simulink model "Vergleich_linear_nichtlinear"  (R2021b)
settings: Solver=FixedStepAuto  StartTime=0.0  StopTime=25  FixedStep=1/1e4  RelTol=1e-3
undefined symbols (not defined in the file): A, B, C, D, S, T_c
settings Model: Creator=basti  LastModifiedBy=basti

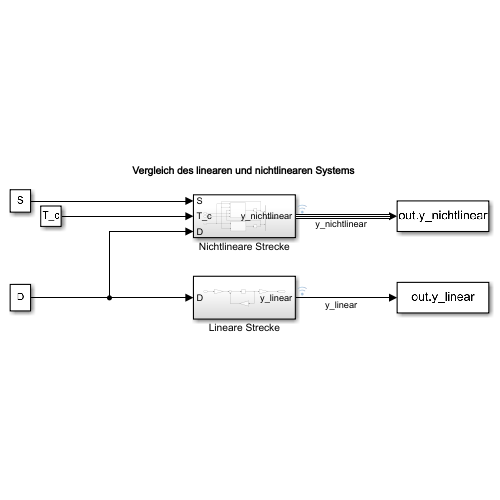
[thumbnail: Simulink's stored preview of the top-level diagram]
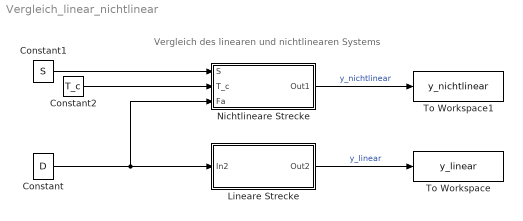
== system Vergleich_linear_nichtlinear ==
  note: Vergleich des linearen und nichtlinearen Systems
  Constant : Constant  Value=D
  Constant1 : Constant  Value=S
  Constant2 : Constant  Value=T_c
  Lineare Strecke : Subsystem
  Nichtlineare Strecke : Subsystem
  To Workspace : ToWorkspace  VariableName=y_linear  SaveFormat=Timeseries  SampleTime=-1
  To Workspace1 : ToWorkspace  VariableName=y_nichtlinear  SaveFormat=Timeseries  SampleTime=-1
  wires:
  Nichtlineare Strecke/1(Out1) -> To Workspace1/1  "y_nichtlinear"
  Lineare Strecke/1(Out2) -> To Workspace/1  "y_linear"
  Constant/1 -> Lineare Strecke/1(In2), Nichtlineare Strecke/3(Fa)
  Constant1/1 -> Nichtlineare Strecke/1(S)
  Constant2/1 -> Nichtlineare Strecke/2(T_c)

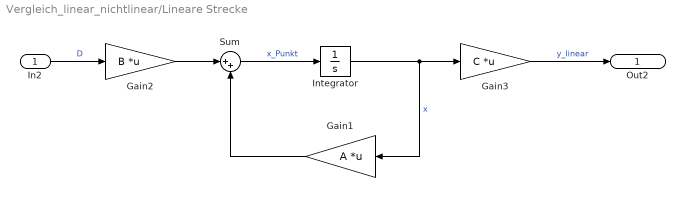
== system Vergleich_linear_nichtlinear/Lineare Strecke ==
  In2 : Inport
  Gain1 : Gain  Gain=A  Multiplication=Matrix(K*u) (u vector)
  Gain2 : Gain  Gain=B  Multiplication=Matrix(K*u) (u vector)
  Gain3 : Gain  Gain=C  Multiplication=Matrix(K*u) (u vector)
  Integrator : Integrator
  Sum : Sum  Inputs=|++
  Out2 : Outport
  wires:
  In2/1 -> Gain2/1  "D"
  Gain2/1 -> Sum/1
  Gain1/1 -> Sum/2
  Sum/1 -> Integrator/1  "x_Punkt"
  Integrator/1 -> Gain3/1, Gain1/1  "x"
  Gain3/1 -> Out2/1  "y_linear"

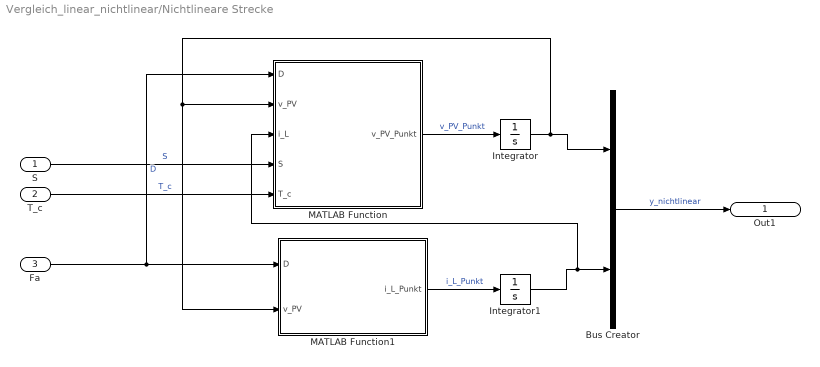
== system Vergleich_linear_nichtlinear/Nichtlineare Strecke ==
  S : Inport
  T_c : Inport  Port=2
  Fa : Inport  Port=3
  Bus Creator : BusCreator  Inputs=2
  Integrator : Integrator
  Integrator1 : Integrator
  MATLAB Function : MATLAB Function  TreatAsAtomicUnit=on
  MATLAB Function1 : MATLAB Function  TreatAsAtomicUnit=on
  Out1 : Outport
  wires:
  MATLAB Function/1(v_PV_Punkt) -> Integrator/1  "v_PV_Punkt"
  MATLAB Function1/1(i_L_Punkt) -> Integrator1/1  "i_L_Punkt"
  Fa/1 -> MATLAB Function/1(D), MATLAB Function1/1(D)  "D"
  Bus Creator/1 -> Out1/1  "y_nichtlinear"
  Integrator1/1 -> MATLAB Function/3(i_L), Bus Creator/2
  Integrator/1 -> MATLAB Function/2(v_PV), MATLAB Function1/2(v_PV), Bus Creator/1
  S/1 -> MATLAB Function/4(S)  "S"
  T_c/1 -> MATLAB Function/5(T_c)  "T_c"

== matlab function Vergleich_linear_nichtlinear/Nichtlineare Strecke/MATLAB Function1 ==
  data: D input; i_L_Punkt output; v_PV input
function i_L_Punkt = fcn(D, v_PV)
    % Konstanten
    c = Konstanten();

    % Berechnung
    i_L_Punkt = 1/c.L * v_PV * D - 1/c.L * c.v_DC;

== matlab function Vergleich_linear_nichtlinear/Nichtlineare Strecke/MATLAB Function ==
  data: D input; v_PV_Punkt output; v_PV input; i_L input; S input; T_c input
function v_PV_Punkt = fcn(D, v_PV, i_L, S, T_c)
    % Konstanten
    c = Konstanten();

    % Berechnung
    i_ph = @(S, T_c) (S/c.S_STC) * c.i_ph_sc_STC * (1 + c.alpha_T * (T_c - c.T_c_STC));             % für Modul
    i_s = @(S, T_c) (i_ph(S, T_c) - (c.v_oc_STC/c.R_h))/(exp(c.v_oc_STC/(c.A_n * c.v_T_STC)) - 1);  % für Modul
    i_d = @(x1, S, T_c) i_s(S, T_c) * (exp(x1/(c.N_s*c.v_T_STC * c.A_n)) - 1);                      % für Modul

    i_pv = @(x1, S, T_c) c.N_p * (i_ph(S, T_c) - i_d(x1, S, T_c) - x1/(c.N_s * c.R_h));

    v_PV_Punkt = 1/c.C * i_pv(v_PV, S, T_c) - 1/c.C * i_L * D;
